simulink model "Animation3D_V20b"  (R2020b)
settings: Solver=VariableStepAuto  StartTime=0.0  StopTime=Sim_t  RelTol=1e-3
libraries: simulink x2, vrlib x1
settings Model: Creator=Mustafa  LastModifiedBy=mustafa
settings DataIOCC: ReturnWorkspaceOutputs=off
settings DebuggingCC: ArithmeticOperatorsInVariantConditions=warning
settings SFSimCC: SimUseLocalCustomCode=off  CustomCodeUndefinedFunction=UseInterfaceOnly
settings RTWCC: RTWUseLocalCustomCode=off
settings CodeAppCC: StateflowObjectComments=on

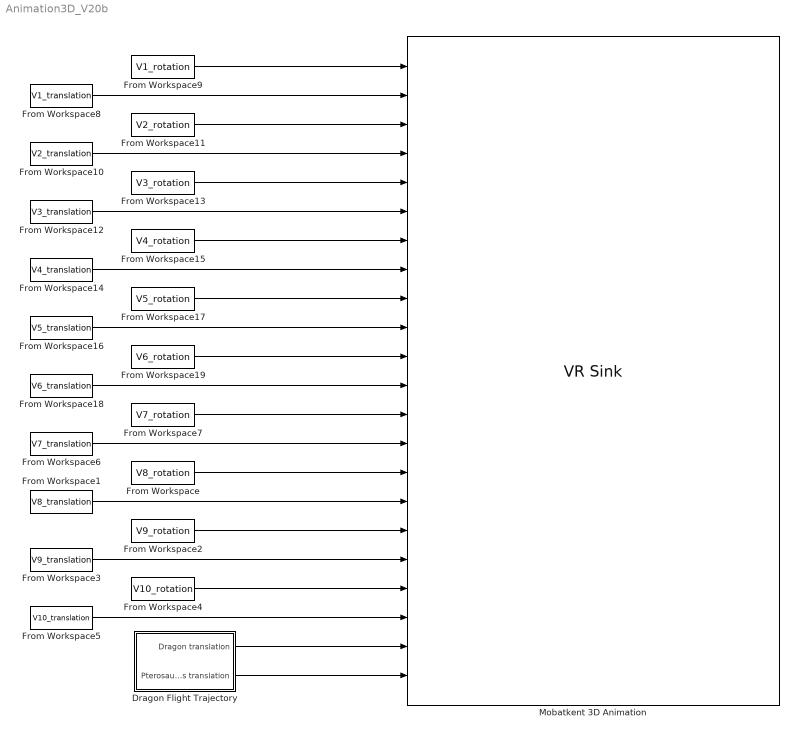
== system Animation3D_V20b ==
  Dragon Flight Trajectory : Subsystem
  From Workspace : FromWorkspace  VariableName=V8_rotation
  From Workspace1 : FromWorkspace  VariableName=V8_translation
  From Workspace10 : FromWorkspace  VariableName=V2_translation
  From Workspace11 : FromWorkspace  VariableName=V2_rotation
  From Workspace12 : FromWorkspace  VariableName=V3_translation
  From Workspace13 : FromWorkspace  VariableName=V3_rotation
  From Workspace14 : FromWorkspace  VariableName=V4_translation
  From Workspace15 : FromWorkspace  VariableName=V4_rotation
  From Workspace16 : FromWorkspace  VariableName=V5_translation
  From Workspace17 : FromWorkspace  VariableName=V5_rotation
  From Workspace18 : FromWorkspace  VariableName=V6_translation
  From Workspace19 : FromWorkspace  VariableName=V6_rotation
  From Workspace2 : FromWorkspace  VariableName=V9_rotation
  From Workspace3 : FromWorkspace  VariableName=V9_translation
  From Workspace4 : FromWorkspace  VariableName=V10_rotation
  From Workspace5 : FromWorkspace  VariableName=V10_translation
  From Workspace6 : FromWorkspace  VariableName=V7_translation
  From Workspace7 : FromWorkspace  VariableName=V7_rotation
  From Workspace8 : FromWorkspace  VariableName=V1_translation
  From Workspace9 : FromWorkspace  VariableName=V1_rotation
  Mobatkent 3D Animation : vrlib/VR Sink  InstantiateOnLoad=on  SampleTime=0.01  ViewEnable=on  RemoteChange=off  RemoteView=off  FieldsWritten=NewCar.rotation.4.1.1.double#NewCar.translation.3.1.1.double#NewCar2.rotation.4.1.1.double#NewCar2.translation.3.1.1.double#NewCar3.rotation.4.1.1.double#NewCar3.translation.3.1.1.double#NewCar4.rotation.4.1.1.double#NewCar4.translation.3.1.1.double#NewCar5.rotation.4.1.1.double#NewCar5.translation.3.1.1.double#NewCar6.rotation.4.1.1.double#NewCar6.translation.3.1.1.double#Car_Mustang.rotation.4.1.1.double#Car_Mustang.translation.3.1.1.double#Fire_Truck.rotation.4.1.1.double#Fire_Truck.translation.3.1.1.double#Car_AR.rotation.4.1.1.double#Car_AR.translation.3.1.1.double#Car_Lotus.rotation.4.1.1.double#Car_Lotus.translation.3.1.1.double#Dragon.translation.3.1.1.double#Pterosaurias.translation.3.1.1.double  WorldFileName=src\Visualization\Mobatkent.WRL  AutoView=on  VideoDimensions=[]  AllowVariableSize=off
  wires:
  From Workspace9/1 -> Mobatkent 3D Animation/1
  From Workspace8/1 -> Mobatkent 3D Animation/2
  From Workspace11/1 -> Mobatkent 3D Animation/3
  From Workspace10/1 -> Mobatkent 3D Animation/4
  From Workspace13/1 -> Mobatkent 3D Animation/5
  From Workspace12/1 -> Mobatkent 3D Animation/6
  From Workspace15/1 -> Mobatkent 3D Animation/7
  From Workspace14/1 -> Mobatkent 3D Animation/8
  From Workspace17/1 -> Mobatkent 3D Animation/9
  From Workspace16/1 -> Mobatkent 3D Animation/10
  From Workspace19/1 -> Mobatkent 3D Animation/11
  From Workspace18/1 -> Mobatkent 3D Animation/12
  From Workspace7/1 -> Mobatkent 3D Animation/13
  From Workspace6/1 -> Mobatkent 3D Animation/14
  From Workspace/1 -> Mobatkent 3D Animation/15
  From Workspace1/1 -> Mobatkent 3D Animation/16
  From Workspace2/1 -> Mobatkent 3D Animation/17
  From Workspace3/1 -> Mobatkent 3D Animation/18
  From Workspace4/1 -> Mobatkent 3D Animation/19
  From Workspace5/1 -> Mobatkent 3D Animation/20
  Dragon Flight Trajectory/1(Dragon translation) -> Mobatkent 3D Animation/21
  Dragon Flight Trajectory/2(Pterosaurias translation) -> Mobatkent 3D Animation/22

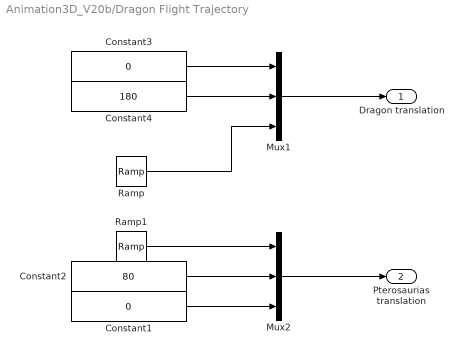
== system Animation3D_V20b/Dragon Flight Trajectory ==
  Constant1 : Constant  Value=0
  Constant2 : Constant  Value=80
  Constant3 : Constant  Value=0
  Constant4 : Constant  Value=180
  Mux1 : Mux  Inputs=3
  Mux2 : Mux  Inputs=3
  Ramp : simulink/Sources/Ramp  slope=40  start=0  InitialOutput=-900
  Ramp1 : simulink/Sources/Ramp  slope=-20  start=0  InitialOutput=700
  Dragon translation : Outport
  Pterosaurias translation : Outport  Port=2
  wires:
  Ramp/1 -> Mux1/3
  Mux1/1 -> Dragon translation/1
  Constant3/1 -> Mux1/1
  Constant4/1 -> Mux1/2
  Constant2/1 -> Mux2/2
  Ramp1/1 -> Mux2/1
  Mux2/1 -> Pterosaurias translation/1
  Constant1/1 -> Mux2/3
